simulink model "SimPrac11"  (R2018a)
settings: Solver=ode45  StartTime=0.0  StopTime=20  RelTol=1e-9
values from neighbouring files (symbols this model uses):
  K2 = 1/Kf    (= 24.2406840555)    [Prac11.m]
  K3 = -1/(K1*Kf)    (= -15865.4906139)    [Prac11.m]
  Kg = Kfg*Kwg*Kag*Rng    [Prac11.m]
  Kr = 1/300    (= 0.00333333333333)    [Prac11.m]
  Ku = 50    [Prac11.m]
  Kusil = 1    [Prac11.m]
  M = Kf*In    (= 0.0115508291498)    [Prac11.m]
  T1 = J/(K1*Kf)    (= 0.00377725600536)    [Prac11.m]
  T1g = Tfg+ Tag    [Prac11.m]
  T2 = (Ta*T1)^0.5    (= 0.00378332483084)    [Prac11.m]
  T2g = (Tfg*Tag)^0.5    [Prac11.m]
  Ta = La/Ra    (= 0.00378940340695)    [Prac11.m]
  Ung = 110    [Prac11.m]
settings Model: Creator=dirlak  LastModifiedBy=dirlak

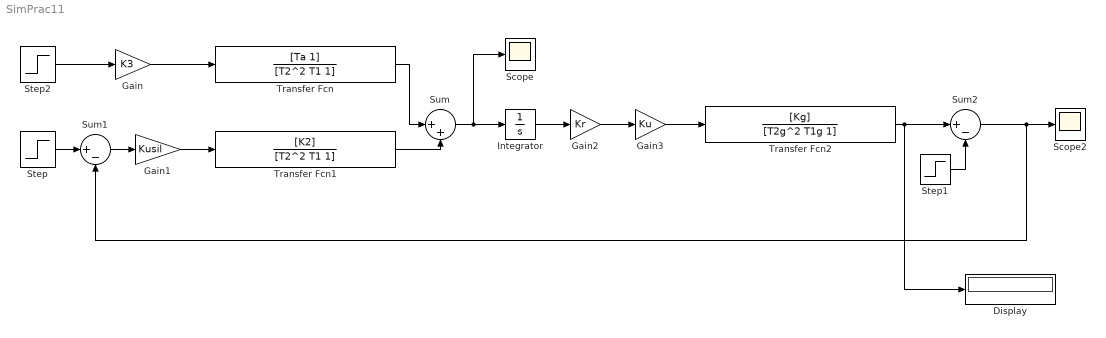
== system SimPrac11 ==
  Display : Display
  Gain : Gain  Gain=K3
  Gain1 : Gain  Gain=Kusil
  Gain2 : Gain  Gain=Kr
  Gain3 : Gain  Gain=Ku
  Integrator : Integrator
  Scope : Scope
  Scope2 : Scope
  Step : Step  Time=0  After=Ung  SampleTime=0
  Step1 : Step  Time=10  After=Ung*0.5  SampleTime=0
  Step2 : Step  Time=0  After=M  SampleTime=0
  Sum : Sum  Inputs=|++
  Sum1 : Sum  Inputs=|+-
  Sum2 : Sum  Inputs=|+-
  Transfer Fcn : TransferFcn  Numerator=[Ta 1]  Denominator=[T2^2 T1 1]
  Transfer Fcn1 : TransferFcn  Numerator=[K2]  Denominator=[T2^2 T1 1]
  Transfer Fcn2 : TransferFcn  Numerator=[Kg]  Denominator=[T2g^2 T1g 1]
  wires:
  Step2/1 -> Gain/1
  Gain/1 -> Transfer Fcn/1
  Transfer Fcn/1 -> Sum/1
  Transfer Fcn1/1 -> Sum/2
  Step/1 -> Sum1/1
  Sum1/1 -> Gain1/1
  Gain1/1 -> Transfer Fcn1/1
  Sum/1 -> Scope/1, Integrator/1
  Integrator/1 -> Gain2/1
  Gain2/1 -> Gain3/1
  Gain3/1 -> Transfer Fcn2/1
  Transfer Fcn2/1 -> Display/1, Sum2/1
  Sum2/1 -> Sum1/2, Scope2/1
  Step1/1 -> Sum2/2
